simulink model "FM_Modulation"  (R2017a)
settings: Solver=VariableStepDiscrete  StartTime=0.0  StopTime=.5  RelTol=1e-3
settings Model: Creator=MohammedHussen  LastModifiedBy=Tahona
settings DataIOCC: LimitDataPoints=on  SaveOutput=off  SaveTime=off
settings OptimizationCC: BooleanDataType=off  DefaultParameterBehavior=Inlined  LocalBlockOutputs=off  LifeSpan=inf
settings DebuggingCC: AlgebraicLoopMsg=error  SingleTaskRateTransMsg=error  AllowSymbolicDim=off  SFUnexpectedBacktrackingDiag=warning  SFNoUnconditionalDefaultTransitionDiag=warning  SFExecutionAtInitializationDiag=none
settings GRTTargetCC: TargetLangStandard=C89/C90 (ANSI)  GeneratePreprocessorConditionals=Disable all
settings ConfigComp: CovMetricSettings=dw  CovHtmlReporting=on  CovSaveCumulativeToWorkspaceVar=on  CovSaveSingleToWorkspaceVar=on  CovExternalEMLEnable=off  CovSFcnEnable=off

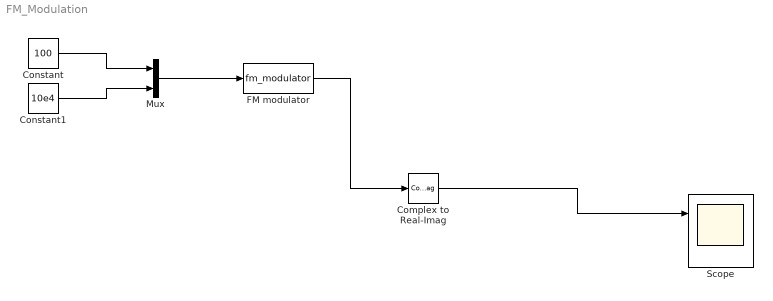
== system FM_Modulation ==
  Complex to Real-Imag : ComplexToRealImag  Output=Real
  Constant : Constant  Value=100
  Constant1 : Constant  Value=10e4
  FM modulator : MATLABFcn  MATLABFcn=fm_modulator
  Mux : Mux  Inputs=2
  Scope : Scope  NumInputPorts=2
  wires:
  FM modulator/1 -> Complex to Real-Imag/1
  Complex to Real-Imag/1 -> Scope/1
  Mux/1 -> FM modulator/1
  Constant/1 -> Mux/1
  Constant1/1 -> Mux/2
